simulink model "testing"  (R2022a)
settings: Solver=VariableStepAuto  StartTime=0.0  StopTime=10.0  RelTol=1e-7
settings Model: Creator=sucho  LastModifiedBy=sucho

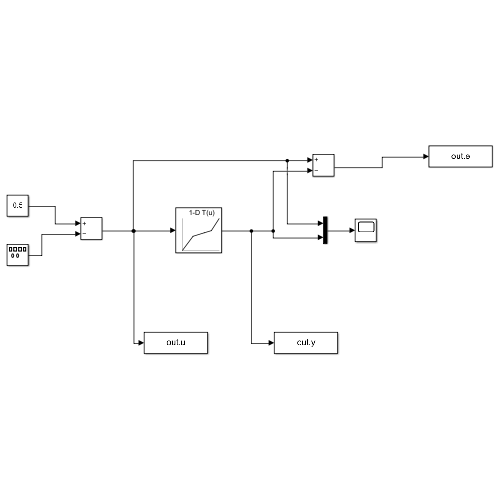
[thumbnail: Simulink's stored preview of the top-level diagram]
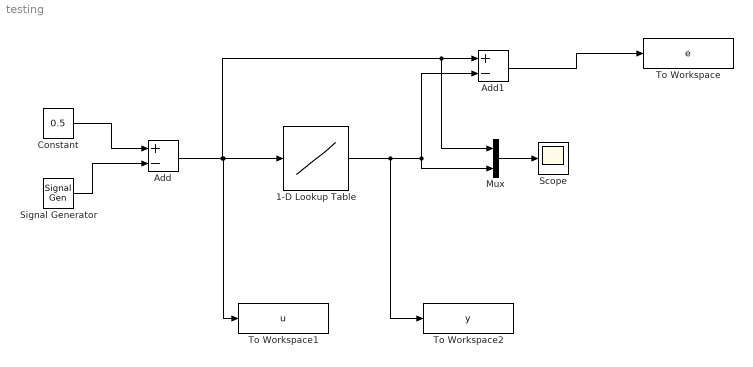
== system testing ==
  1-D Lookup Table : Lookup_n-D  NumberOfTableDimensions=1  BreakpointsForDimension1=[-0 0.3 0.6 0.8 1]  Table=[3 7 8 8.5 12]  InternalRulePriority=Speed  RndMeth=Simplest
  Add : Sum  Inputs=+-
  Add1 : Sum  Inputs=+-
  Constant : Constant  Value=0.5
  Mux : Mux  Inputs=2
  Scope : Scope
  Signal Generator : SignalGenerator  Amplitude=0.5  Units=rad/sec
  To Workspace : ToWorkspace  VariableName=e  SaveFormat=Timeseries  SampleTime=0.1
  To Workspace1 : ToWorkspace  VariableName=u  SaveFormat=Timeseries  SampleTime=0.1
  To Workspace2 : ToWorkspace  VariableName=y  SaveFormat=Timeseries  SampleTime=0.1
      settings: Save2DSignal=2-D array (concatenate along first dimension)
  wires:
  Constant/1 -> Add/1
  Signal Generator/1 -> Add/2
  Add/1 -> Mux/1, Add1/1, To Workspace1/1, 1-D Lookup Table/1
  1-D Lookup Table/1 -> To Workspace2/1, Add1/2, Mux/2
  Mux/1 -> Scope/1
  Add1/1 -> To Workspace/1
